simulink model "Model1_3_ZVD"  (R2021a)
settings: Solver=VariableStepAuto  StartTime=0.0  StopTime=20  RelTol=1e-3
InitFcn:
  | ml=2;
  | 
  | mc=0.5;
  | M2=0.5;
  | 
  | mt=5;
  | g=9.81;
  | l_ref=0.1;
  | l_ini=1;
  | l=l_ini;
  | x_ref=1;
  | n1=5;n2=1;
  | 
  | %ADRC' s parameter caculation
  | %b0 = (ml+mc)/(mc*ml +mc*mt+ml*mt); %Hieu
  | b0=(ml+mc)/(mt*mc+2*ml*mc+mt*ml+ml^2+mc^2); %Enhanced-coupling
  | k_ESO = 100;
  | T_set  = 6;
  | 
  | s_cl = -5.85/T_set;
  | Kp   = s_cl^2;
  | Kd   = -2*s_cl;
  | 
  | s_ESO = k_ESO*s_cl;
  | l1        = -3*s_ESO;
  | l2        = 3*( s_ESO)^2;
  | l3        = -(s_ESO)^3;
  | 
  | %b1 = (mt+mc)/(mc*ml +mc*mt+ml*mt);
  | b1=1/(ml+mc);
  | k_ESO1 =100;
  | T_set1  = 3;
  | s_cl1 = -5.85/T_set1;
  | Kp1   = s_cl1^2;
  | Kd1   = -2*s_cl1;
  | 
  | s_ESO1 = k_ESO1*s_cl1;
  | l11        = -3*s_ESO1;
  | l21        = 3*( s_ESO1)^2;
  | l31        = -(s_ESO1)^3;
  | 
  | 
  | L1=l_ini;
  | %L2=0.5;
  | L2=0.1;
  | m1=2;
  | m2=mc;
  | m=5;
  | %Bo input shaping
  | alpha = (1/L1 + 1/L2)*(m1+M2)/m1;
  | beta = (((m1+M2)/m1)^2)*((1/L1 + 1/L2)^2) - 4*(m1+M2)/(m1*L1*L2);
  | w1 = sqrt(g*(alpha - sqrt(beta))/2);
  | w2 = sqrt(g*(alpha + sqrt(beta))/2);
  | damping_ratio = 0;
  | wd1 = w1*sqrt(1-damping_ratio^2);
  | wd2 = w2*sqrt(1-damping_ratio^2);
  | k = exp(damping_ratio*pi/sqrt(1-damping_ratio^2));
  | 
  | %ZVD1
  | t1_ZVD_1=pi/wd1;
  | ... (+27 lines)
values from neighbouring files (symbols this model uses):
  particle = repmat(empty_particle, nPop, 1)    [PSO16_12.m]    (also in PSO_ZVD.m)
undefined symbols (not defined in the file or in its folder): E1_tt, E2_tt, E3_tt, i, li, xi
libraries: neural x66, simulink_extras x4, simulink x2
(part 15 of 20)

== matlab function Model1_3_ZVD/RBF_ZVD_m=5_m1=1/enhanced3/Crane ==
  data: dx1 output; d1x input; l1 input; d1l1 input; the1 input; d1the1 input; the2 input; d1the2 input; Fx input; Fl input; dx2 output; dx3 output; dx4 output; dx5 output; dx6 output; m2 input; dx7 output; dx8 output
function [dx1,dx2,dx3,dx4,dx5,dx6,dx7,dx8] = fcn(d1x,l1,d1l1,the1,d1the1,the2,d1the2,Fx,Fl,m2)
 m =5; m1 =2; g =9.81; l2=0.5;bx=25; bl=50;bc=0.1;

 dx1=d1x;

 dx2 = (Fx*l1*l2*m2*cos(the1 - the2)^2 - Fx*l1*l2*m2 - d1the2^2*l1*l2^2*m2^2*sin(the2) - Fx*l1*l2*m1 + Fx*l1*l2*m2*sin(the1 - the2)^2 + bx*d1x*l1*l2*m1 + bx*d1x*l1*l2*m2 + Fl*l1*l2*m1*sin(the1) + Fl*l1*l2*m2*sin(the1) - bc*d1the1*l2*m1*cos(the1) - bc*d1the1*l2*m2*cos(the1) - bc*d1the2*l1*m1*cos(the2) - bc*d1the2*l1*m2*cos(the2) + bc*d1the2*l1*m1*sin(the1 - the2)*sin(the1) + bc*d1the2*l1*m2*sin(the1 - the2)*sin(the1) + d1the2^2*l1*l2^2*m2^2*cos(the1 - the2)*sin(the1) - d1the2^2*l1*l2^2*m2^2*sin(the1 - the2)*cos(the1) - d1the2^2*l1*l2^2*m1*m2*sin(the2) - g*l1*l2*m2^2*cos(the2)*sin(the2) - Fl*l1*l2*m2*cos(the1 - the2)^2*sin(the1) + bc*d1the1*l2*m2*sin(the1 - the2)^2*cos(the1) - bl*d1l1*l1*l2*m1*sin(the1) - bl*d1l1*l1*l2*m2*sin(the1) + d1the2^2*l1*l2^2*m2^2*cos(the1 - the2)^2*sin(the2) - d1the2^2*l1*l2^2*m2^2*cos(the1 - the2)^3*sin(the1) + d1the2^2*l1*l2^2*m2^2*sin(the1 - the2)^3*cos(the1) + d1the2^2*l1*l2^2*m2^2*sin(the1 - the2)^2*sin(the2) - bx*d1x*l1*l2*m2*cos(the1 - the2)^2 - Fl*l1*l2*m2*sin(the1 - the2)*cos(the2) + bc*d1the2*l1*m1*cos(the1 - the2)*cos(the1) + bc*d1the2*l1*m2*cos(the1 - the2)*cos(the1) + bc*d1the1*l2*m2*cos(the1 - the2)*cos(the2) - bx*d1x*l1*l2*m2*sin(the1 - the2)^2 - bc*d1the1*l2*m2*cos(the1 - the2)*sin(the1 - the2)*sin(the1) + d1the2^2*l1*l2^2*m1*m2*cos(the1 - the2)*sin(the1) - d1the2^2*l1*l2^2*m1*m2*sin(the1 - the2)*cos(the1) + g*l1*l2*m2^2*cos(the1 - the2)*cos(the1)*sin(the2) + g*l1*l2*m2^2*cos(the1 - the2)*cos(the2)*sin(the1) - g*l1*l2*m2^2*sin(the1 - the2)*cos(the1)*cos(the2) - g*l1*l2*m1*m2*cos(the2)*sin(the2) + g*l1*l2*m2^2*sin(the1 - the2)*sin(the1)*sin(the2) + bl*d1l1*l1*l2*m2*sin(the1 - the2)*cos(the2) + d1the2^2*l1*l2^2*m2^2*cos(the1 - the2)^2*sin(the1 - the2)*cos(the1) - d1the2^2*l1*l2^2*m2^2*cos(the1 - the2)*sin(the1 - the2)^2*sin(the1) - g*l1*l2*m2^2*cos(the1 - the2)^2*cos(the1)*sin(the1) + g*l1*l2*m2^2*sin(the1 - the2)^2*cos(the1)*sin(the1) + bl*d1l1*l1*l2*m2*cos(the1 - the2)^2*sin(the1) + g*l1*l2*m2^2*cos(the1 - the2)*sin(the1 - the2)*cos(the1)^2 - g*l1*l2*m2^2*cos(the1 - the2)*sin(the1 - the2)*sin(the1)^2 + Fl*l1*l2*m2*cos(the1 - the2)*sin(the1 - the2)*cos(the1) + g*l1*l2*m1*m2*cos(the1 - the2)*cos(the1)*sin(the2) + g*l1*l2*m1*m2*cos(the1 - the2)*cos(the2)*sin(the1) - g*l1*l2*m1*m2*sin(the1 - the2)*cos(the1)*cos(the2) + g*l1*l2*m1*m2*sin(the1 - the2)*sin(the1)*sin(the2) - bl*d1l1*l1*l2*m2*cos(the1 - the2)*sin(the1 - the2)*cos(the1) - g*l1*l2*m1*m2*cos(the1 - the2)^2*cos(the1)*sin(the1) + g*l1*l2*m1*m2*sin(the1 - the2)^2*cos(the1)*sin(the1) + g*l1*l2*m1*m2*cos(the1 - the2)*sin(the1 - the2)*cos(the1)^2 - g*l1*l2*m1*m2*cos(the1 - the2)*sin(the1 - the2)*sin(the1)^2)/(l1*l2*(m1^2*cos(the1)^2 - m*m2 - 2*m1*m2 - m*m1 + m2^2*cos(the1)^2 + m2^2*cos(the2)^2 + m1^2*sin(the1)^2 + m2^2*sin(the1)^2 + m2^2*cos(the1 - the2)^2 + m2^2*sin(the1 - the2)^2 - m1^2 - m2^2 + 2*m1*m2*cos(the1)^2 + m1*m2*cos(the2)^2 + 2*m1*m2*sin(the1)^2 + m*m2*cos(the1 - the2)^2 + m1*m2*cos(the1 - the2)^2 + m*m2*sin(the1 - the2)^2 + m1*m2*sin(the1 - the2)^2 - m2^2*cos(the1 - the2)^2*sin(the1)^2 - m2^2*sin(the1 - the2)^2*cos(the1)^2 - 2*m2^2*sin(the1 - the2)*cos(the2)*sin(the1) - 2*m2^2*cos(the1 - the2)*cos(the1)*cos(the2) - m1*m2*cos(the1 - the2)^2*sin(the1)^2 - m1*m2*sin(the1 - the2)^2*cos(the1)^2 + 2*m2^2*cos(the1 - the2)*sin(the1 - the2)*cos(the1)*sin(the1) - 2*m1*m2*sin(the1 - the2)*cos(the2)*sin(the1) - 2*m1*m2*cos(the1 - the2)*cos(the1)*cos(the2) + 2*m1*m2*cos(the1 - the2)*sin(the1 - the2)*cos(the1)*sin(the1)));

 dx3=d1l1;

 dx4 = (Fx*l1*l2*m1^2*sin(the1) - d1the1^2*l1^2*l2*m2^3 - Fl*l1*l2*m1^2 - Fl*l1*l2*m2^2 - d1the2^2*l1*l2^2*m2^3*cos(the1 - the2) - d1the1^2*l1^2*l2*m1^3 + Fx*l1*l2*m2^2*sin(the1) - g*l1*l2*m1^3*cos(the1) - g*l1*l2*m2^3*cos(the1) - Fl*l1*l2*m*m1 - Fl*l1*l2*m*m2 - 2*Fl*l1*l2*m1*m2 + d1the1^2*l1^2*l2*m1^3*cos(the1)^2 + d1the1^2*l1^2*l2*m2^3*cos(the1)^2 + d1the1^2*l1^2*l2*m2^3*cos(the2)^2 + d1the1^2*l1^2*l2*m1^3*sin(the1)^2 + d1the1^2*l1^2*l2*m2^3*sin(the1)^2 - bc*d1the2*l1*m1^2*sin(the1 - the2) - bc*d1the2*l1*m2^2*sin(the1 - the2) + Fl*l1*l2*m1^2*cos(the1)^2 + Fl*l1*l2*m2^2*cos(the1)^2 + Fl*l1*l2*m2^2*cos(the2)^2 + d1the1^2*l1^2*l2*m2^3*cos(the1 - the2)^2 + d1the2^2*l1*l2^2*m2^3*cos(the1 - the2)^3 - d1the1^2*l1^2*l2*m*m1^2 - d1the1^2*l1^2*l2*m*m2^2 - 3*d1the1^2*l1^2*l2*m1*m2^2 - 3*d1the1^2*l1^2*l2*m1^2*m2 + d1the1^2*l1^2*l2*m2^3*sin(the1 - the2)^2 + g*l1*l2*m1^3*cos(the1)^3 + g*l1*l2*m2^3*cos(the1)^3 + Fl*l1*l2*m2^2*cos(the1 - the2)^2 + bl*d1l1*l1*l2*m1^2 + bl*d1l1*l1*l2*m2^2 - bl*d1l1*l1*l2*m1^2*cos(the1)^2 - bl*d1l1*l1*l2*m2^2*cos(the1)^2 - bl*d1l1*l1*l2*m2^2*cos(the2)^2 + d1the1^2*l1^2*l2*m*m2^2*sin(the1 - the2)^2 + 2*d1the1^2*l1^2*l2*m1*m2^2*sin(the1 - the2)^2 + d1the1^2*l1^2*l2*m1^2*m2*sin(the1 - the2)^2 + 3*g*l1*l2*m1*m2^2*cos(the1)^3 + 3*g*l1*l2*m1^2*m2*cos(the1)^3 + bc*d1the1*l2*m1^2*cos(the1)*sin(the1) + bc*d1the1*l2*m2^2*cos(the1)*sin(the1) + bc*d1the2*l1*m1^2*cos(the2)*sin(the1) + bc*d1the2*l1*m2^2*cos(the2)*sin(the1) - bl*d1l1*l1*l2*m2^2*cos(the1 - the2)^2 - Fx*l1*l2*m2^2*sin(the1 - the2)*cos(the2) + 2*Fx*l1*l2*m1*m2*sin(the1) + d1the2^2*l1*l2^2*m2^3*cos(the1 - the2)*cos(the1)^2 + d1the2^2*l1*l2^2*m2^3*cos(the1 - the2)*cos(the2)^2 - g*l1*l2*m2^3*sin(the1 - the2)*sin(the2) + g*l1*l2*m2^3*cos(the1)*cos(the2)^2 + bc*d1the1*l2*m2^2*cos(the1 - the2)*sin(the1 - the2) - bc*d1the2*l1*m*m1*sin(the1 - the2) - bc*d1the2*l1*m*m2*sin(the1 - the2) - 2*bc*d1the2*l1*m1*m2*sin(the1 - the2) + g*l1*l2*m1^3*cos(the1)*sin(the1)^2 + g*l1*l2*m2^3*cos(the1)*sin(the1)^2 + 2*Fl*l1*l2*m1*m2*cos(the1)^2 + Fl*l1*l2*m1*m2*cos(the2)^2 - Fx*l1*l2*m2^2*cos(the1 - the2)^2*sin(the1) - d1the2^2*l1*l2^2*m*m2^2*cos(the1 - the2) - 2*d1the2^2*l1*l2^2*m1*m2^2*cos(the1 - the2) - d1the2^2*l1*l2^2*m1^2*m2*cos(the1 - the2) - 2*d1the1^2*l1^2*l2*m*m1*m2 + d1the2^2*l1*l2^2*m2^3*cos(the1 - the2)*sin(the1 - the2)^2 + g*l1*l2*m2^3*cos(the1 - the2)^2*cos(the1) - g*l1*l2*m*m1^2*cos(the1) - g*l1*l2*m*m2^2*cos(the1) - 3*g*l1*l2*m1*m2^2*cos(the1) - 3*g*l1*l2*m1^2*m2*cos(the1) + bc*d1the2*l1*m1^2*sin(the1 - the2)*cos(the1)^2 + bc*d1the2*l1*m2^2*sin(the1 - the2)*cos(the1)^2 - bx*d1x*l1*l2*m1^2*sin(the1) - bx*d1x*l1*l2*m2^2*sin(the1) + Fl*l1*l2*m*m2*cos(the1 - the2)^2 + Fl*l1*l2*m1*m2*cos(the1 - the2)^2 + 3*d1the1^2*l1^2*l2*m1*m2^2*cos(the1)^2 + 3*d1the1^2*l1^2*l2*m1^2*m2*cos(the1)^2 + 2*d1the1^2*l1^2*l2*m1*m2^2*cos(the2)^2 + d1the1^2*l1^2*l2*m1^2*m2*cos(the2)^2 + bl*d1l1*l1*l2*m*m1 + bl*d1l1*l1*l2*m*m2 + 2*bl*d1l1*l1*l2*m1*m2 - d1the1^2*l1^2*l2*m2^3*cos(the1 - the2)^2*sin(the1)^2 - d1the1^2*l1^2*l2*m2^3*sin(the1 - the2)^2*cos(the1)^2 + 3*d1the1^2*l1^2*l2*m1*m2^2*sin(the1)^2 + 3*d1the1^2*l1^2*l2*m1^2*m2*sin(the1)^2 + d1the2^2*l1*l2^2*m2^3*sin(the1)*sin(the2) + d1the1^2*l1^2*l2*m*m2^2*cos(the1 - the2)^2 + 2*d1the1^2*l1^2*l2*m1*m2^2*cos(the1 - the2)^2 + d1the1^2*l1^2*l2*m1^2*m2*cos(the1 - the2)^2 + d1the2^2*l1*l2^2*m*m2^2*cos(the1 - the2)^3 + d1the2^2*l1*l2^2*m1*m2^2*cos(the1 - the2)^3 - 2*d1the1^2*l1^2*l2*m2^3*sin(the1 - the2)*cos(the2)*sin(the1) + d1the2^2*l1*l2^2*m2^3*sin(the1 - the2)*cos(the1)*sin(the1) - d1the2^2*l1*l2^2*m2^3*sin(the1 - the2)*cos(the2)*sin(the2) - 2*Fl*l1*l2*m2^2*cos(the1 - the2)*cos(the1)*cos(the2) + d1the1^2*l1^2*l2*m*m1*m2*cos(the1 - the2)^2 - 2*bl*d1l1*l1*l2*m1*m2*cos(the1)^2 - bl*d1l1*l1*l2*m1*m2*cos(the2)^2 + g*l1*l2*m2^3*cos(the2)*sin(the1)*sin(the2) + d1the2^2*l1*l2^2*m*m2^2*cos(the1 - the2)*sin(the1 - the2)^2 + d1the2^2*l1*l2^2*m1*m2^2*cos(the1 - the2)*sin(the1 - the2)^2 + g*l1*l2*m*m2^2*cos(the1 - the2)^2*cos(the1) + 2*g*l1*l2*m1*m2^2*cos(the1 - the2)^2*cos(the1) + g*l1*l2*m1^2*m2*cos(the1 - the2)^2*cos(the1) + d1the1^2*l1^2*l2*m*m1*m2*sin(the1 - the2)^2 + bx*d1x*l1*l2*m2^2*cos(the1 - the2)^2*sin(the1) - bc*d1the2*l1*m1^2*cos(the1 - the2)*cos(the1)*sin(the1) - bc*d1the2*l1*m2^2*cos(the1 - the2)*cos(the1)*sin(the1) - bc*d1the1*l2*m2^2*cos(the1 - the2)*cos(the2)*sin(the1) - bc*d1the1*l2*m2^2*sin(the1 - the2)*cos(the1)*cos(the2) + 2*bc*d1the1*l2*m1*m2*cos(the1)*sin(the1) + 2*bc*d1the2*l1*m1*m2*cos(the2)*sin(the1) - 2*d1the2^2*l1*l2^2*m2^3*cos(the1 - the2)^2*cos(the1)*cos(the2) - bl*d1l1*l1*l2*m*m2*cos(the1 - the2)^2 - bl*d1l1*l1*l2*m1*m2*cos(the1 - the2)^2 - 2*d1the1^2*l1^2*l2*m1*m2^2*cos(the1 - the2)^2*sin(the1)^2 - 2*d1the1^2*l1^2*l2*m1*m2^2*sin(the1 - the2)^2*cos(the1)^2 - d1the1^2*l1^2*l2*m1^2*m2*cos(the1 - the2)^2*sin(the1)^2 - d1the1^2*l1^2*l2*m1^2*m2*sin(the1 - the2)^2*cos(the1)^2 + Fx*l1*l2*m2^2*cos(the1 - the2)*sin(the1 - the2)*cos(the1) - Fx*l1*l2*m1*m2*sin(the1 - the2)*cos(the2) - d1the2^2*l1*l2^2*m2^3*sin(the1 - the2)^2*cos(the1)*cos(the2) - d1the2^2*l1*l2^2*m2^3*cos(the1 - the2)^2*sin(the1)*sin(the2) + 2*d1the2^2*l1*l2^2*m1*m2^2*sin(the1)*sin(the2) + d1the2^2*l1*l2^2*m1^2*m2*sin(the1)*sin(the2) + g*l1*l2*m2^3*cos(the1 - the2)*sin(the1 - the2)*sin(the1) - 2*g*l1*l2*m2^3*cos(the1 - the2)*cos(the1)^2*cos(the2) + bc*d1the1*l2*m*m2*cos(the1 - the2)*sin(the1 - the2) + bc*d1the1*l2*m1*m2*cos(the1 - the2)*sin(the1 - the2) - g*l1*l2*m2^3*cos(the1 - the2)*cos(the2)*sin(the1)^2 + g*l1*l2*m2^3*sin(the1 - the2)*cos(the1)^2*sin(the2) - Fx*l1*l2*m1*m2*cos(the1 - the2)^2*sin(the1) - d1the2^2*l1*l2^2*m*m1*m2*cos(the1 - the2) - 2*g*l1*l2*m*m1*m2*cos(the1) + bx*d1x*l1*l2*m2^2*sin(the1 - the2)*cos(the2) + 2*bc*d1the2*l1*m1*m2*sin(the1 - the2)*cos(the1)^2 - 2*bx*d1x*l1*l2*m1*m2*sin(the1) + 2*d1the2^2*l1*l2^2*m1*m2^2*cos(the1 - the2)*cos(the1)^2 + d1the2^2*l1*l2^2*m1^2*m2*cos(the1 - the2)*cos(the1)^2 + d1the2^2*l1*l2^2*m1*m2^2*cos(the1 - the2)*cos(the2)^2 - g*l1*l2*m*m2^2*sin(the1 - the2)*sin(the2) - 2*g*l1*l2*m1*m2^2*sin(the1 - the2)*sin(the2) - g*l1*l2*m1^2*m2*sin(the1 - the2)*sin(the2) - 2*d1the1^2*l1^2*l2*m2^3*cos(the1 - the2)*cos(the1)*cos(the2) + 2*g*l1*l2*m1*m2^2*cos(the1)*cos(the2)^2 + g*l1*l2*m1^2*m2*cos(the1)*cos(the2)^2 + 3*g*l1*l2*m1*m2^2*cos(the1)*sin(the1)^2 + 3*g*l1*l2*m1^2*m2*cos(the1)*sin(the1)^2 - 2*g*l1*l2*m1*m2^2*cos(the1 - the2)*cos(the2)*sin(the1)^2 - g*l1*l2*m1^2*m2*cos(the1 - the2)*cos(the2)*sin(the1)^2 + 2*d1the1^2*l1^2*l2*m2^3*cos(the1 - the2)*sin(the1 - the2)*cos(the1)*sin(the1) + d1the2^2*l1*l2^2*m2^3*cos(the1 - the2)*sin(the1 - the2)*cos(the1)*sin(the2) - d1the2^2*l1*l2^2*m2^3*cos(the1 - the2)*sin(the1 - the2)*cos(the2)*sin(the1) + 2*g*l1*l2*m1*m2^2*sin(the1 - the2)*cos(the1)^2*sin(the2) + g*l1*l2*m1^2*m2*sin(the1 - the2)*cos(the1)^2*sin(the2) - 2*Fl*l1*l2*m1*m2*cos(the1 - the2)*cos(the1)*cos(the2) - g*l1*l2*m2^3*cos(the1 - the2)*cos(the1)*sin(the1)*sin(the2) - g*l1*l2*m2^3*sin(the1 - the2)*cos(the1)*cos(the2)*sin(the1) + g*l1*l2*m*m1*m2*cos(the1 - the2)^2*cos(the1) + bx*d1x*l1*l2*m1*m2*cos(the1 - the2)^2*sin(the1) - 2*bc*d1the2*l1*m1*m2*cos(the1 - the2)*cos(the1)*sin(the1) - bc*d1the1*l2*m1*m2*cos(the1 - the2)*cos(the2)*sin(the1) - bc*d1the1*l2*m1*m2*sin(the1 - the2)*cos(the1)*cos(the2) - 4*d1the1^2*l1^2*l2*m1*m2^2*cos(the1 - the2)*cos(the1)*cos(the2) - 2*d1the1^2*l1^2*l2*m1^2*m2*cos(the1 - the2)*cos(the1)*cos(the2) + Fx*l1*l2*m1*m2*cos(the1 - the2)*sin(the1 - the2)*cos(the1) - 4*d1the1^2*l1^2*l2*m1*m2^2*sin(the1 - the2)*cos(the2)*sin(the1) - 2*d1the1^2*l1^2*l2*m1^2*m2*sin(the1 - the2)*cos(the2)*sin(the1) + 2*d1the2^2*l1*l2^2*m1*m2^2*sin(the1 - the2)*cos(the1)*sin(the1) + d1the2^2*l1*l2^2*m1^2*m2*sin(the1 - the2)*cos(the1)*sin(the1) - d1the2^2*l1*l2^2*m1*m2^2*sin(the1 - the2)*cos(the2)*sin(the2) + 2*g*l1*l2*m1*m2^2*cos(the2)*sin(the1)*sin(the2) + g*l1*l2*m1^2*m2*cos(the2)*sin(the1)*sin(the2) + 2*bl*d1l1*l1*l2*m2^2*cos(the1 - the2)*cos(the1)*cos(the2) - 2*d1the2^2*l1*l2^2*m1*m2^2*cos(the1 - the2)^2*cos(the1)*cos(the2) - d1the2^2*l1*l2^2*m1*m2^2*sin(the1 - the2)^2*cos(the1)*cos(the2) - bx*d1x*l1*l2*m2^2*cos(the1 - the2)*sin(the1 - the2)*cos(the1) + bx*d1x*l1*l2*m1*m2*sin(the1 - the2)*cos(the2) - d1the2^2*l1*l2^2*m1*m2^2*cos(the1 - the2)^2*sin(the1)*sin(the2) + g*l1*l2*m*m2^2*cos(the1 - the2)*sin(the1 - the2)*sin(the1) + 2*g*l1*l2*m1*m2^2*cos(the1 - the2)*sin(the1 - the2)*sin(the1) + g*l1*l2*m1^2*m2*cos(the1 - the2)*sin(the1 - the2)*sin(the1) - g*l1*l2*m*m1*m2*sin(the1 - the2)*sin(the2) - 4*g*l1*l2*m1*m2^2*cos(the1 - the2)*cos(the1)^2*cos(the2) - 2*g*l1*l2*m1^2*m2*cos(the1 - the2)*cos(the1)^2*cos(the2) + 4*d1the1^2*l1^2*l2*m1*m2^2*cos(the1 - the2)*sin(the1 - the2)*cos(the1)*sin(the1) + 2*d1the1^2*l1^2*l2*m1^2*m2*cos(the1 - the2)*sin(the1 - the2)*cos(the1)*sin(the1) + d1the2^2*l1*l2^2*m1*m2^2*cos(the1 - the2)*sin(the1 - the2)*cos(the1)*sin(the2) - d1the2^2*l1*l2^2*m1*m2^2*cos(the1 - the2)*sin(the1 - the2)*cos(the2)*sin(the1) - 2*g*l1*l2*m1*m2^2*cos(the1 - the2)*cos(the1)*sin(the1)*sin(the2) - 2*g*l1*l2*m1*m2^2*sin(the1 - the2)*cos(the1)*cos(the2)*sin(the1) - g*l1*l2*m1^2*m2*cos(the1 - the2)*cos(the1)*sin(the1)*sin(the2) - g*l1*l2*m1^2*m2*sin(the1 - the2)*cos(the1)*cos(the2)*sin(the1) + 2*bl*d1l1*l1*l2*m1*m2*cos(the1 - the2)*cos(the1)*cos(the2) - bx*d1x*l1*l2*m1*m2*cos(the1 - the2)*sin(the1 - the2)*cos(the1) + g*l1*l2*m*m1*m2*cos(the1 - the2)*sin(the1 - the2)*sin(the1))/(l1*l2*(m1 + m2)*(m1^2*cos(the1)^2 - m*m2 - 2*m1*m2 - m*m1 + m2^2*cos(the1)^2 + m2^2*cos(the2)^2 + m1^2*sin(the1)^2 + m2^2*sin(the1)^2 + m2^2*cos(the1 - the2)^2 + m2^2*sin(the1 - the2)^2 - m1^2 - m2^2 + 2*m1*m2*cos(the1)^2 + m1*m2*cos(the2)^2 + 2*m1*m2*sin(the1)^2 + m*m2*cos(the1 - the2)^2 + m1*m2*cos(the1 - the2)^2 + m*m2*sin(the1 - the2)^2 + m1*m2*sin(the1 - the2)^2 - m2^2*cos(the1 - the2)^2*sin(the1)^2 - m2^2*sin(the1 - the2)^2*cos(the1)^2 - 2*m2^2*sin(the1 - the2)*cos(the2)*sin(the1) - 2*m2^2*cos(the1 - the2)*cos(the1)*cos(the2) - m1*m2*cos(the1 - the2)^2*sin(the1)^2 - m1*m2*sin(the1 - the2)^2*cos(the1)^2 + 2*m2^2*cos(the1 - the2)*sin(the1 - the2)*cos(the1)*sin(the1) - 2*m1*m2*sin(the1 - the2)*cos(the2)*sin(the1) - 2*m1*m2*cos(the1 - the2)*cos(the1)*cos(the2) + 2*m1*m2*cos(the1 - the2)*sin(the1 - the2)*cos(the1)*sin(the1)));
 
 dx5=d1the1;

 dx6 = -(bc*d1the2*l1*m1^2*cos(the1 - the2) - bc*d1the1*l2*m2^2 - Fx*l1*l2*m1^2*cos(the1) - Fx*l1*l2*m2^2*cos(the1) - d1the2^2*l1*l2^2*m2^3*sin(the1 - the2) - g*l1*l2*m1^3*sin(the1) - g*l1*l2*m2^3*sin(the1) - bc*d1the1*l2*m1^2 + bc*d1the2*l1*m2^2*cos(the1 - the2) - bc*d1the1*l2*m*m1 - bc*d1the1*l2*m*m2 - 2*bc*d1the1*l2*m1*m2 + bc*d1the1*l2*m2^2*cos(the2)^2 + d1the2^2*l1*l2^2*m2^3*sin(the1 - the2)^3 + bc*d1the1*l2*m1^2*sin(the1)^2 + bc*d1the1*l2*m2^2*sin(the1)^2 + g*l1*l2*m1^3*sin(the1)^3 + g*l1*l2*m2^3*sin(the1)^3 - 2*d1l1*d1the1*l1*l2*m1^3 - 2*d1l1*d1the1*l1*l2*m2^3 + bc*d1the1*l2*m2^2*sin(the1 - the2)^2 + 2*d1l1*d1the1*l1*l2*m1^3*cos(the1)^2 + 2*d1l1*d1the1*l1*l2*m2^3*cos(the1)^2 + 2*d1l1*d1the1*l1*l2*m2^3*cos(the2)^2 + Fl*l1*l2*m1^2*cos(the1)*sin(the1) + Fl*l1*l2*m2^2*cos(the1)*sin(the1) - bc*d1the2*l1*m1^2*cos(the1)*cos(the2) - bc*d1the2*l1*m2^2*cos(the1)*cos(the2) + d1the2^2*l1*l2^2*m*m2^2*sin(the1 - the2)^3 + d1the2^2*l1*l2^2*m1*m2^2*sin(the1 - the2)^3 + 2*d1l1*d1the1*l1*l2*m1^3*sin(the1)^2 + 2*d1l1*d1the1*l1*l2*m2^3*sin(the1)^2 + 3*g*l1*l2*m1*m2^2*sin(the1)^3 + 3*g*l1*l2*m1^2*m2*sin(the1)^3 + Fx*l1*l2*m2^2*cos(the1 - the2)*cos(the2) - 2*Fx*l1*l2*m1*m2*cos(the1) + 2*d1l1*d1the1*l1*l2*m2^3*cos(the1 - the2)^2 - 2*d1l1*d1the1*l1*l2*m*m1^2 - 2*d1l1*d1the1*l1*l2*m*m2^2 - 6*d1l1*d1the1*l1*l2*m1*m2^2 - 6*d1l1*d1the1*l1*l2*m1^2*m2 + 2*d1l1*d1the1*l1*l2*m2^3*sin(the1 - the2)^2 + g*l1*l2*m2^3*cos(the1 - the2)*sin(the2) + Fl*l1*l2*m2^2*cos(the1 - the2)*sin(the1 - the2) + bc*d1the2*l1*m*m1*cos(the1 - the2) + bc*d1the2*l1*m*m2*cos(the1 - the2) + 2*bc*d1the2*l1*m1*m2*cos(the1 - the2) + d1the2^2*l1*l2^2*m2^3*sin(the1 - the2)*cos(the2)^2 + d1the2^2*l1*l2^2*m2^3*sin(the1 - the2)*sin(the1)^2 + g*l1*l2*m1^3*cos(the1)^2*sin(the1) + g*l1*l2*m2^3*cos(the1)^2*sin(the1) + g*l1*l2*m2^3*cos(the2)^2*sin(the1) + Fx*l1*l2*m2^2*sin(the1 - the2)^2*cos(the1) + bx*d1x*l1*l2*m1^2*cos(the1) + bx*d1x*l1*l2*m2^2*cos(the1) + bc*d1the1*l2*m1*m2*cos(the2)^2 + d1the2^2*l1*l2^2*m2^3*cos(the1 - the2)^2*sin(the1 - the2) - d1the2^2*l1*l2^2*m*m2^2*sin(the1 - the2) - 2*d1the2^2*l1*l2^2*m1*m2^2*sin(the1 - the2) - d1the2^2*l1*l2^2*m1^2*m2*sin(the1 - the2) - bc*d1the2*l1*m1^2*cos(the1 - the2)*sin(the1)^2 - bc*d1the2*l1*m2^2*cos(the1 - the2)*sin(the1)^2 + 2*bc*d1the1*l2*m1*m2*sin(the1)^2 - g*l1*l2*m*m1^2*sin(the1) - g*l1*l2*m*m2^2*sin(the1) - 3*g*l1*l2*m1*m2^2*sin(the1) - 3*g*l1*l2*m1^2*m2*sin(the1) + g*l1*l2*m2^3*sin(the1 - the2)^2*sin(the1) + bc*d1the1*l2*m*m2*sin(the1 - the2)^2 + bc*d1the1*l2*m1*m2*sin(the1 - the2)^2 - d1the2^2*l1*l2^2*m2^3*cos(the1)*sin(the2) - g*l1*l2*m2^3*cos(the1)*cos(the2)*sin(the2) - Fl*l1*l2*m2^2*cos(the1 - the2)*cos(the2)*sin(the1) - Fl*l1*l2*m2^2*sin(the1 - the2)*cos(the1)*cos(the2) + 2*Fl*l1*l2*m1*m2*cos(the1)*sin(the1) + d1the2^2*l1*l2^2*m*m2^2*cos(the1 - the2)^2*sin(the1 - the2) + d1the2^2*l1*l2^2*m1*m2^2*cos(the1 - the2)^2*sin(the1 - the2) - 2*bc*d1the2*l1*m1*m2*cos(the1)*cos(the2) - bx*d1x*l1*l2*m2^2*sin(the1 - the2)^2*cos(the1) + bc*d1the2*l1*m1^2*sin(the1 - the2)*cos(the1)*sin(the1) + bc*d1the2*l1*m2^2*sin(the1 - the2)*cos(the1)*sin(the1) - 2*bc*d1the1*l2*m2^2*sin(the1 - the2)*cos(the2)*sin(the1) + g*l1*l2*m*m2^2*sin(the1 - the2)^2*sin(the1) + 2*g*l1*l2*m1*m2^2*sin(the1 - the2)^2*sin(the1) + g*l1*l2*m1^2*m2*sin(the1 - the2)^2*sin(the1) + Fx*l1*l2*m1*m2*cos(the1 - the2)*cos(the2) - 4*d1l1*d1the1*l1*l2*m*m1*m2 - d1the2^2*l1*l2^2*m2^3*cos(the1 - the2)^2*cos(the2)*sin(the1) - 2*d1the2^2*l1*l2^2*m1*m2^2*cos(the1)*sin(the2) - d1the2^2*l1*l2^2*m1^2*m2*cos(the1)*sin(the2) - Fx*l1*l2*m2^2*cos(the1 - the2)*sin(the1 - the2)*sin(the1) + d1the2^2*l1*l2^2*m2^3*sin(the1 - the2)^2*cos(the1)*sin(the2) - 2*d1the2^2*l1*l2^2*m2^3*sin(the1 - the2)^2*cos(the2)*sin(the1) + g*l1*l2*m2^3*cos(the1 - the2)*sin(the1 - the2)*cos(the1) + 6*d1l1*d1the1*l1*l2*m1*m2^2*cos(the1)^2 + 6*d1l1*d1the1*l1*l2*m1^2*m2*cos(the1)^2 + 4*d1l1*d1the1*l1*l2*m1*m2^2*cos(the2)^2 + 2*d1l1*d1the1*l1*l2*m1^2*m2*cos(the2)^2 - 2*d1l1*d1the1*l1*l2*m2^3*cos(the1 - the2)^2*sin(the1)^2 - 2*d1l1*d1the1*l1*l2*m2^3*sin(the1 - the2)^2*cos(the1)^2 + Fl*l1*l2*m*m2*cos(the1 - the2)*sin(the1 - the2) + Fl*l1*l2*m1*m2*cos(the1 - the2)*sin(the1 - the2) + 6*d1l1*d1the1*l1*l2*m1*m2^2*sin(the1)^2 + 6*d1l1*d1the1*l1*l2*m1^2*m2*sin(the1)^2 - bl*d1l1*l1*l2*m1^2*cos(the1)*sin(the1) - bl*d1l1*l1*l2*m2^2*cos(the1)*sin(the1) - g*l1*l2*m2^3*sin(the1 - the2)*cos(the1)^2*cos(the2) + 2*d1l1*d1the1*l1*l2*m*m2^2*cos(the1 - the2)^2 + 4*d1l1*d1the1*l1*l2*m1*m2^2*cos(the1 - the2)^2 + 2*d1l1*d1the1*l1*l2*m1^2*m2*cos(the1 - the2)^2 - g*l1*l2*m2^3*cos(the1 - the2)*sin(the1)^2*sin(the2) - 2*g*l1*l2*m2^3*sin(the1 - the2)*cos(the2)*sin(the1)^2 + Fx*l1*l2*m1*m2*sin(the1 - the2)^2*cos(the1) - bx*d1x*l1*l2*m2^2*cos(the1 - the2)*cos(the2) + 2*bx*d1x*l1*l2*m1*m2*cos(the1) + 2*d1l1*d1the1*l1*l2*m*m2^2*sin(the1 - the2)^2 + 4*d1l1*d1the1*l1*l2*m1*m2^2*sin(the1 - the2)^2 + 2*d1l1*d1the1*l1*l2*m1^2*m2*sin(the1 - the2)^2 - d1the2^2*l1*l2^2*m*m1*m2*sin(the1 - the2) - 2*bc*d1the2*l1*m1*m2*cos(the1 - the2)*sin(the1)^2 + g*l1*l2*m*m2^2*cos(the1 - the2)*sin(the2) + 2*g*l1*l2*m1*m2^2*cos(the1 - the2)*sin(the2) + g*l1*l2*m1^2*m2*cos(the1 - the2)*sin(the2) - 2*g*l1*l2*m*m1*m2*sin(the1) + d1the2^2*l1*l2^2*m1*m2^2*sin(the1 - the2)*cos(the2)^2 - bl*d1l1*l1*l2*m2^2*cos(the1 - the2)*sin(the1 - the2) + d1the2^2*l1*l2^2*m2^3*cos(the1 - the2)*cos(the1)*sin(the1) + d1the2^2*l1*l2^2*m2^3*cos(the1 - the2)*cos(the2)*sin(the2) + 2*d1the2^2*l1*l2^2*m1*m2^2*sin(the1 - the2)*sin(the1)^2 + d1the2^2*l1*l2^2*m1^2*m2*sin(the1 - the2)*sin(the1)^2 + 3*g*l1*l2*m1*m2^2*cos(the1)^2*sin(the1) + 3*g*l1*l2*m1^2*m2*cos(the1)^2*sin(the1) + 2*g*l1*l2*m1*m2^2*cos(the2)^2*sin(the1) + g*l1*l2*m1^2*m2*cos(the2)^2*sin(the1) - 2*g*l1*l2*m1*m2^2*sin(the1 - the2)*cos(the1)^2*cos(the2) - g*l1*l2*m1^2*m2*sin(the1 - the2)*cos(the1)^2*cos(the2) - g*l1*l2*m2^3*cos(the1 - the2)*cos(the1)*cos(the2)*sin(the1) - 2*g*l1*l2*m1*m2^2*cos(the1 - the2)*sin(the1)^2*sin(the2) - 4*g*l1*l2*m1*m2^2*sin(the1 - the2)*cos(the2)*sin(the1)^2 - g*l1*l2*m1^2*m2*cos(the1 - the2)*sin(the1)^2*sin(the2) - 2*g*l1*l2*m1^2*m2*sin(the1 - the2)*cos(the2)*sin(the1)^2 - d1the2^2*l1*l2^2*m2^3*cos(the1 - the2)*sin(the1 - the2)*sin(the1)*sin(the2) - Fl*l1*l2*m1*m2*cos(the1 - the2)*cos(the2)*sin(the1) - Fl*l1*l2*m1*m2*sin(the1 - the2)*cos(the1)*cos(the2) - bx*d1x*l1*l2*m1*m2*sin(the1 - the2)^2*cos(the1) + g*l1*l2*m2^3*sin(the1 - the2)*cos(the1)*sin(the1)*sin(the2) + 2*bc*d1the2*l1*m1*m2*sin(the1 - the2)*cos(the1)*sin(the1) - 2*bc*d1the1*l2*m1*m2*sin(the1 - the2)*cos(the2)*sin(the1) + g*l1*l2*m*m1*m2*sin(the1 - the2)^2*sin(the1) + 2*d1the2^2*l1*l2^2*m1*m2^2*cos(the1 - the2)*cos(the1)*sin(the1) + d1the2^2*l1*l2^2*m1^2*m2*cos(the1 - the2)*cos(the1)*sin(the1) + d1the2^2*l1*l2^2*m1*m2^2*cos(the1 - the2)*cos(the2)*sin(the2) - Fx*l1*l2*m1*m2*cos(the1 - the2)*sin(the1 - the2)*sin(the1) - 2*g*l1*l2*m1*m2^2*cos(the1)*cos(the2)*sin(the2) - g*l1*l2*m1^2*m2*cos(the1)*cos(the2)*sin(the2) - 4*d1l1*d1the1*l1*l2*m2^3*cos(the1 - the2)*cos(the1)*cos(the2) + bl*d1l1*l1*l2*m2^2*cos(the1 - the2)*cos(the2)*sin(the1) + bl*d1l1*l1*l2*m2^2*sin(the1 - the2)*cos(the1)*cos(the2) - 2*bl*d1l1*l1*l2*m1*m2*cos(the1)*sin(the1) - 4*d1l1*d1the1*l1*l2*m2^3*sin(the1 - the2)*cos(the2)*sin(the1) + 2*d1l1*d1the1*l1*l2*m*m1*m2*cos(the1 - the2)^2 - bx*d1x*l1*l2*m1*m2*cos(the1 - the2)*cos(the2) - d1the2^2*l1*l2^2*m1*m2^2*cos(the1 - the2)^2*cos(the2)*sin(the1) + 2*d1l1*d1the1*l1*l2*m*m1*m2*sin(the1 - the2)^2 + d1the2^2*l1*l2^2*m1*m2^2*sin(the1 - the2)^2*cos(the1)*sin(the2) - 2*d1the2^2*l1*l2^2*m1*m2^2*sin(the1 - the2)^2*cos(the2)*sin(the1) + g*l1*l2*m*m2^2*cos(the1 - the2)*sin(the1 - the2)*cos(the1) + 2*g*l1*l2*m1*m2^2*cos(the1 - the2)*sin(the1 - the2)*cos(the1) + g*l1*l2*m1^2*m2*cos(the1 - the2)*sin(the1 - the2)*cos(the1) + g*l1*l2*m*m1*m2*cos(the1 - the2)*sin(the2) + bx*d1x*l1*l2*m2^2*cos(the1 - the2)*sin(the1 - the2)*sin(the1) - 4*d1l1*d1the1*l1*l2*m1*m2^2*cos(the1 - the2)^2*sin(the1)^2 - 4*d1l1*d1the1*l1*l2*m1*m2^2*sin(the1 - the2)^2*cos(the1)^2 - 2*d1l1*d1the1*l1*l2*m1^2*m2*cos(the1 - the2)^2*sin(the1)^2 - 2*d1l1*d1the1*l1*l2*m1^2*m2*sin(the1 - the2)^2*cos(the1)^2 - d1the2^2*l1*l2^2*m2^3*cos(the1 - the2)*sin(the1 - the2)*cos(the1)*cos(the2) - bl*d1l1*l1*l2*m*m2*cos(the1 - the2)*sin(the1 - the2) - bl*d1l1*l1*l2*m1*m2*cos(the1 - the2)*sin(the1 - the2) - 8*d1l1*d1the1*l1*l2*m1*m2^2*sin(the1 - the2)*cos(the2)*sin(the1) - 4*d1l1*d1the1*l1*l2*m1^2*m2*sin(the1 - the2)*cos(the2)*sin(the1) - d1the2^2*l1*l2^2*m1*m2^2*cos(the1 - the2)*sin(the1 - the2)*cos(the1)*cos(the2) - 2*g*l1*l2*m1*m2^2*cos(the1 - the2)*cos(the1)*cos(the2)*sin(the1) - g*l1*l2*m1^2*m2*cos(the1 - the2)*cos(the1)*cos(the2)*sin(the1) - d1the2^2*l1*l2^2*m1*m2^2*cos(the1 - the2)*sin(the1 - the2)*sin(the1)*sin(the2) + 2*g*l1*l2*m1*m2^2*sin(the1 - the2)*cos(the1)*sin(the1)*sin(the2) + g*l1*l2*m1^2*m2*sin(the1 - the2)*cos(the1)*sin(the1)*sin(the2) + bl*d1l1*l1*l2*m1*m2*cos(the1 - the2)*cos(the2)*sin(the1) + bl*d1l1*l1*l2*m1*m2*sin(the1 - the2)*cos(the1)*cos(the2) + 4*d1l1*d1the1*l1*l2*m2^3*cos(the1 - the2)*sin(the1 - the2)*cos(the1)*sin(the1) + g*l1*l2*m*m1*m2*cos(the1 - the2)*sin(the1 - the2)*cos(the1) + bx*d1x*l1*l2*m1*m2*cos(the1 - the2)*sin(the1 - the2)*sin(the1) - 8*d1l1*d1the1*l1*l2*m1*m2^2*cos(the1 - the2)*cos(the1)*cos(the2) - 4*d1l1*d1the1*l1*l2*m1^2*m2*cos(the1 - the2)*cos(the1)*cos(the2) + 8*d1l1*d1the1*l1*l2*m1*m2^2*cos(the1 - the2)*sin(the1 - the2)*cos(the1)*sin(the1) + 4*d1l1*d1the1*l1*l2*m1^2*m2*cos(the1 - the2)*sin(the1 - the2)*cos(the1)*sin(the1))/(l1^2*l2*(m1 + m2)*(m1^2*cos(the1)^2 - m*m2 - 2*m1*m2 - m*m1 + m2^2*cos(the1)^2 + m2^2*cos(the2)^2 + m1^2*sin(the1)^2 + m2^2*sin(the1)^2 + m2^2*cos(the1 - the2)^2 + m2^2*sin(the1 - the2)^2 - m1^2 - m2^2 + 2*m1*m2*cos(the1)^2 + m1*m2*cos(the2)^2 + 2*m1*m2*sin(the1)^2 + m*m2*cos(the1 - the2)^2 + m1*m2*cos(the1 - the2)^2 + m*m2*sin(the1 - the2)^2 + m1*m2*sin(the1 - the2)^2 - m2^2*cos(the1 - the2)^2*sin(the1)^2 - m2^2*sin(the1 - the2)^2*cos(the1)^2 - 2*m2^2*sin(the1 - the2)*cos(the2)*sin(the1) - 2*m2^2*cos(the1 - the2)*cos(the1)*cos(the2) - m1*m2*cos(the1 - the2)^2*sin(the1)^2 - m1*m2*sin(the1 - the2)^2*cos(the1)^2 + 2*m2^2*cos(the1 - the2)*sin(the1 - the2)*cos(the1)*sin(the1) - 2*m1*m2*sin(the1 - the2)*cos(the2)*sin(the1) - 2*m1*m2*cos(the1 - the2)*cos(the1)*cos(the2) + 2*m1*m2*cos(the1 - the2)*sin(the1 - the2)*cos(the1)*sin(the1)));

 dx7=d1the2;

 dx8 = -(bc*d1the1*l2*m2^2*cos(the1 - the2) - bc*d1the2*l1*m2^2 - Fx*l1*l2*m2^2*cos(the2) - g*l1*l2*m2^3*sin(the2) - Fl*l1*l2*m2^2*sin(the1 - the2) - bc*d1the2*l1*m1^2 - bc*d1the2*l1*m*m1 - bc*d1the2*l1*m*m2 - 2*bc*d1the2*l1*m1*m2 + bc*d1the2*l1*m1^2*cos(the1)^2 + bc*d1the2*l1*m2^2*cos(the1)^2 + bc*d1the2*l1*m1^2*sin(the1)^2 + bc*d1the2*l1*m2^2*sin(the1)^2 + Fl*l1*l2*m2^2*cos(the2)*sin(the1) - bc*d1the1*l2*m2^2*cos(the1)*cos(the2) + Fx*l1*l2*m2^2*cos(the1 - the2)*cos(the1) - Fx*l1*l2*m1*m2*cos(the2) + Fx*l1*l2*m2^2*sin(the1 - the2)*sin(the1) + g*l1*l2*m2^3*cos(the1 - the2)*sin(the1) - g*l1*l2*m2^3*sin(the1 - the2)*cos(the1) - Fl*l1*l2*m*m2*sin(the1 - the2) - Fl*l1*l2*m1*m2*sin(the1 - the2) + bc*d1the1*l2*m*m2*cos(the1 - the2) + bc*d1the1*l2*m1*m2*cos(the1 - the2) + g*l1*l2*m2^3*cos(the1)^2*sin(the2) + g*l1*l2*m2^3*sin(the1)^2*sin(the2) + Fl*l1*l2*m2^2*sin(the1 - the2)*cos(the1)^2 + bx*d1x*l1*l2*m2^2*cos(the2) + 2*bc*d1the2*l1*m1*m2*cos(the1)^2 - bc*d1the1*l2*m2^2*cos(the1 - the2)*sin(the1)^2 + 2*bc*d1the2*l1*m1*m2*sin(the1)^2 - g*l1*l2*m2^3*cos(the1 - the2)*sin(the1)^3 + g*l1*l2*m2^3*sin(the1 - the2)*cos(the1)^3 - g*l1*l2*m*m2^2*sin(the2) - 2*g*l1*l2*m1*m2^2*sin(the2) - g*l1*l2*m1^2*m2*sin(the2) + bl*d1l1*l1*l2*m2^2*sin(the1 - the2) - d1the2^2*l1*l2^2*m2^3*cos(the2)*sin(the2) + 2*g*l1*l2*m1*m2^2*sin(the1)^2*sin(the2) + g*l1*l2*m1^2*m2*sin(the1)^2*sin(the2) + d1the2^2*l1*l2^2*m2^3*sin(the1 - the2)*sin(the1)*sin(the2) - Fl*l1*l2*m2^2*cos(the1 - the2)*cos(the1)*sin(the1) + Fl*l1*l2*m1*m2*cos(the2)*sin(the1) - bc*d1the1*l2*m1*m2*cos(the1)*cos(the2) - bl*d1l1*l1*l2*m2^2*sin(the1 - the2)*cos(the1)^2 - 2*g*l1*l2*m1*m2^2*cos(the1 - the2)*sin(the1)^3 + 2*g*l1*l2*m1*m2^2*sin(the1 - the2)*cos(the1)^3 - g*l1*l2*m1^2*m2*cos(the1 - the2)*sin(the1)^3 + g*l1*l2*m1^2*m2*sin(the1 - the2)*cos(the1)^3 + bc*d1the1*l2*m2^2*sin(the1 - the2)*cos(the1)*sin(the1) + Fx*l1*l2*m1*m2*cos(the1 - the2)*cos(the1) - d1the2^2*l1*l2^2*m2^3*cos(the1 - the2)^2*cos(the1)*sin(the1) - d1the2^2*l1*l2^2*m1*m2^2*cos(the2)*sin(the2) + Fx*l1*l2*m1*m2*sin(the1 - the2)*sin(the1) + d1the2^2*l1*l2^2*m2^3*sin(the1 - the2)^2*cos(the1)*sin(the1) + d1the2^2*l1*l2^2*m2^3*cos(the1 - the2)*sin(the1 - the2)*cos(the1)^2 - bl*d1l1*l1*l2*m2^2*cos(the2)*sin(the1) - d1the2^2*l1*l2^2*m2^3*cos(the1 - the2)*sin(the1 - the2)*sin(the1)^2 - g*l1*l2*m2^3*cos(the1 - the2)*cos(the1)^2*sin(the1) + g*l1*l2*m2^3*sin(the1 - the2)*cos(the1)*sin(the1)^2 + Fl*l1*l2*m1*m2*sin(the1 - the2)*cos(the1)^2 - bx*d1x*l1*l2*m2^2*cos(the1 - the2)*cos(the1) + bx*d1x*l1*l2*m1*m2*cos(the2) - bc*d1the1*l2*m1*m2*cos(the1 - the2)*sin(the1)^2 + g*l1*l2*m*m2^2*cos(the1 - the2)*sin(the1) - g*l1*l2*m*m2^2*sin(the1 - the2)*cos(the1) + 2*g*l1*l2*m1*m2^2*cos(the1 - the2)*sin(the1) - 2*g*l1*l2*m1*m2^2*sin(the1 - the2)*cos(the1) + g*l1*l2*m1^2*m2*cos(the1 - the2)*sin(the1) - g*l1*l2*m1^2*m2*sin(the1 - the2)*cos(the1) - g*l1*l2*m*m1*m2*sin(the2) - bx*d1x*l1*l2*m2^2*sin(the1 - the2)*sin(the1) + d1the2^2*l1*l2^2*m2^3*cos(the1 - the2)*cos(the1)*sin(the2) + d1the2^2*l1*l2^2*m2^3*cos(the1 - the2)*cos(the2)*sin(the1) - d1the2^2*l1*l2^2*m2^3*sin(the1 - the2)*cos(the1)*cos(the2) + bl*d1l1*l1*l2*m*m2*sin(the1 - the2) + bl*d1l1*l1*l2*m1*m2*sin(the1 - the2) + 2*g*l1*l2*m1*m2^2*cos(the1)^2*sin(the2) + g*l1*l2*m1^2*m2*cos(the1)^2*sin(the2) - d1the2^2*l1*l2^2*m1*m2^2*cos(the1 - the2)*sin(the1 - the2)*sin(the1)^2 - 2*g*l1*l2*m1*m2^2*cos(the1 - the2)*cos(the1)^2*sin(the1) - g*l1*l2*m1^2*m2*cos(the1 - the2)*cos(the1)^2*sin(the1) + 2*g*l1*l2*m1*m2^2*sin(the1 - the2)*cos(the1)*sin(the1)^2 + g*l1*l2*m1^2*m2*sin(the1 - the2)*cos(the1)*sin(the1)^2 - Fl*l1*l2*m1*m2*cos(the1 - the2)*cos(the1)*sin(the1) - bl*d1l1*l1*l2*m1*m2*sin(the1 - the2)*cos(the1)^2 + bc*d1the1*l2*m1*m2*sin(the1 - the2)*cos(the1)*sin(the1) + d1the2^2*l1*l2^2*m1*m2^2*cos(the1 - the2)*cos(the1)*sin(the2) + d1the2^2*l1*l2^2*m1*m2^2*cos(the1 - the2)*cos(the2)*sin(the1) - d1the2^2*l1*l2^2*m1*m2^2*sin(the1 - the2)*cos(the1)*cos(the2) + d1the2^2*l1*l2^2*m1*m2^2*sin(the1 - the2)*sin(the1)*sin(the2) + bl*d1l1*l1*l2*m2^2*cos(the1 - the2)*cos(the1)*sin(the1) - bl*d1l1*l1*l2*m1*m2*cos(the2)*sin(the1) - bx*d1x*l1*l2*m1*m2*cos(the1 - the2)*cos(the1) - d1the2^2*l1*l2^2*m1*m2^2*cos(the1 - the2)^2*cos(the1)*sin(the1) + d1the2^2*l1*l2^2*m1*m2^2*sin(the1 - the2)^2*cos(the1)*sin(the1) + g*l1*l2*m*m1*m2*cos(the1 - the2)*sin(the1) - g*l1*l2*m*m1*m2*sin(the1 - the2)*cos(the1) - bx*d1x*l1*l2*m1*m2*sin(the1 - the2)*sin(the1) + d1the2^2*l1*l2^2*m1*m2^2*cos(the1 - the2)*sin(the1 - the2)*cos(the1)^2 + bl*d1l1*l1*l2*m1*m2*cos(the1 - the2)*cos(the1)*sin(the1))/(l1*l2^2*m2*(m1^2*cos(the1)^2 - m*m2 - 2*m1*m2 - m*m1 + m2^2*cos(the1)^2 + m2^2*cos(the2)^2 + m1^2*sin(the1)^2 + m2^2*sin(the1)^2 + m2^2*cos(the1 - the2)^2 + m2^2*sin(the1 - the2)^2 - m1^2 - m2^2 + 2*m1*m2*cos(the1)^2 + m1*m2*cos(the2)^2 + 2*m1*m2*sin(the1)^2 + m*m2*cos(the1 - the2)^2 + m1*m2*cos(the1 - the2)^2 + m*m2*sin(the1 - the2)^2 + m1*m2*sin(the1 - the2)^2 - m2^2*cos(the1 - the2)^2*sin(the1)^2 - m2^2*sin(the1 - the2)^2*cos(the1)^2 - 2*m2^2*sin(the1 - the2)*cos(the2)*sin(the1) - 2*m2^2*cos(the1 - the2)*cos(the1)*cos(the2) - m1*m2*cos(the1 - the2)^2*sin(the1)^2 - m1*m2*sin(the1 - the2)^2*cos(the1)^2 + 2*m2^2*cos(the1 - the2)*sin(the1 - the2)*cos(the1)*sin(the1) - 2*m1*m2*sin(the1 - the2)*cos(the2)*sin(the1) - 2*m1*m2*cos(the1 - the2)*cos(the1)*cos(the2) + 2*m1*m2*cos(the1 - the2)*sin(the1 - the2)*cos(the1)*sin(the1)));
